simulink model "realtime_maglev_model"  (R2013a)
settings: Solver=ode45  StartTime=0.0  StopTime=10.0  RelTol=1e-3
undefined symbols (not defined in the file or in its folder): Advantech, PCI
libraries: rtwinlib x2, simulink x2
settings Model: Creator=Levitador  LastModifiedBy=Levitador

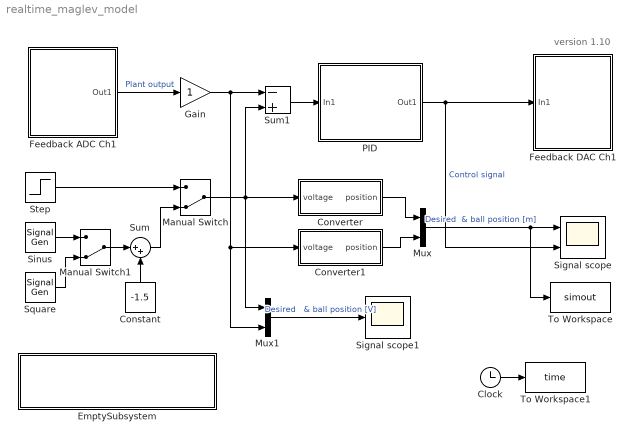
== system realtime_maglev_model ==
  note: version 1.10
  Clock : Clock
  Constant : Constant  Value=-1.5
  Converter : Subsystem
  Converter1 : Subsystem
  EmptySubsystem : Subsystem
      mask Display:
      | image(imread('FB-inst-blue2.jpg'))
      | disp('\n\nFeedback Instruments Limited')
  Feedback ADC Ch1 : Subsystem  mask{Tsamp=0.001}
      mask prompts: Tsamp "Sampling time"
      mask Display:
      | image(imread('bckg.bmp'))
      | disp('PCI1711 \n Lab I/O Board \n\n Feedback  ADC')
  Feedback DAC Ch1 : Subsystem  mask(DAC Unit for Feedback Experiments){st=0.001, ch=1}
      mask prompts: st "Sample Time"; ch "Output Channel"
      mask help:
      | Digital to Analog Output  for Feedback Experiments
      | using Advantech PCI1711  I/O board
      mask Display:
      | image(imread('bckg.bmp'))
      | disp('PCI1711 \n Lab I/O Board \n\n Feedback  DAC')
  Gain : Gain
  Manual Switch : ManualSwitch  CurrentSetting=0
  Manual Switch1 : ManualSwitch  CurrentSetting=0
  Mux : Mux  Inputs=2
  Mux1 : Mux  Inputs=2
  PID : Subsystem  mask{Kp=4, Ki=2.3, Kd=0.2}
      mask Display:
      | image(imread('bckg.bmp'))
      | disp('PID')
  Signal scope : Scope  NumInputPorts=2
      settings: TimeRange=100  YMin=0.0135~-175  YMax=0.0215~175  MaxDataPoints=500000
      mask Display: image(imread('scope.jpg'))
  Signal scope1 : Scope
      settings: TimeRange=100  YMin=-2.4  YMax=-0.7  MaxDataPoints=500000
      mask Display: image(imread('scope.jpg'))
  Sinus : SignalGenerator  Amplitude=0.5  Frequency=0.5
  Square : SignalGenerator  WaveForm=square  Amplitude=0.4  Frequency=0.1
  Step : Step  Time=10  Before=-1  After=-2  SampleTime=0
  Sum : Sum  Inputs=|++
  Sum1 : Sum  Inputs=-+  SaturateOnIntegerOverflow=on  InputSameDT=on  OutDataTypeStr=Inherit: Same as first input
  To Workspace : ToWorkspace  VariableName=simout  SampleTime=0.01
  To Workspace1 : ToWorkspace  VariableName=time  SampleTime=0.01
  wires:
  Sum1/1 -> PID/1(In1)
  Feedback ADC Ch1/1(Out1) -> Gain/1  "Plant output"
  PID/1(Out1) -> Feedback DAC Ch1/1(In1), Signal scope/2  "Control signal"
  Step/1 -> Manual Switch/1
  Square/1 -> Manual Switch1/2
  Sinus/1 -> Manual Switch1/1
  Manual Switch/1 -> Sum1/2, Converter/1(voltage), Mux1/1
  Manual Switch1/1 -> Sum/1
  Constant/1 -> Sum/2
  Sum/1 -> Manual Switch/2
  Mux/1 -> Signal scope/1, To Workspace/1  "Desired  & ball position [m]"
  Converter/1(position) -> Mux/1
  Converter1/1(position) -> Mux/2
  Mux1/1 -> Signal scope1/1  "Desired   & ball position [V]"
  Clock/1 -> To Workspace1/1
  Gain/1 -> Sum1/1, Converter1/1(voltage), Mux1/2

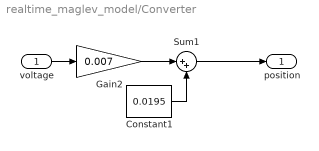
== system realtime_maglev_model/Converter ==
  voltage : Inport
  Constant1 : Constant  Value=0.0195
  Gain2 : Gain  Gain=0.007
  Sum1 : Sum  Inputs=|++
  position : Outport
  wires:
  Gain2/1 -> Sum1/1
  Constant1/1 -> Sum1/2
  voltage/1 -> Gain2/1
  Sum1/1 -> position/1

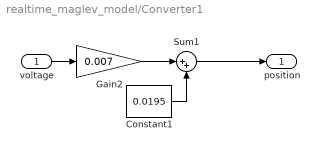
== system realtime_maglev_model/Converter1 ==
  voltage : Inport
  Constant1 : Constant  Value=0.0195
  Gain2 : Gain  Gain=0.007
  Sum1 : Sum  Inputs=|++
  position : Outport
  wires:
  Sum1/1 -> position/1
  voltage/1 -> Gain2/1
  Constant1/1 -> Sum1/2
  Gain2/1 -> Sum1/1

== system realtime_maglev_model/EmptySubsystem ==

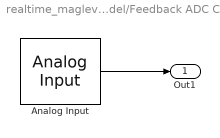
== system realtime_maglev_model/Feedback ADC Ch1 ==
  Analog Input : rtwinlib/Analog Input  SampleTime=Tsamp  MaxMissedTicks=10  ShowMissedTicks=off  YieldWhenWaiting=off  DrvName=Advantech/PCI-1711  DrvAddress=4294967295  DrvOptions=zeros(1,0)  Channels=11  RangeMode=1  VoltRange=1  DataType=1
      settings: AttributesFormatString=Advantech\nPCI-1711 [auto]
  Out1 : Outport
  wires:
  Analog Input/1 -> Out1/1

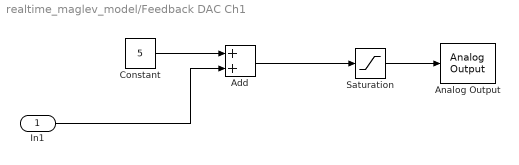
== system realtime_maglev_model/Feedback DAC Ch1 ==
  In1 : Inport
  Add : Sum  OutDataTypeStr=Inherit: Same as first input
  Analog Output : rtwinlib/Analog Output  SampleTime=st  MaxMissedTicks=10  ShowMissedTicks=off  YieldWhenWaiting=off  DrvName=Advantech/PCI-1711  DrvAddress=4294967295  DrvOptions=zeros(1,0)  Channels=ch  RangeMode=1  VoltRange=2  InitialValue=5  FinalValue=5
      settings: AttributesFormatString=Advantech\nPCI-1711 [auto]
  Constant : Constant  Value=5
  Saturation : Saturate  UpperLimit=10  LowerLimit=0
  wires:
  In1/1 -> Add/2
  Constant/1 -> Add/1
  Saturation/1 -> Analog Output/1
  Add/1 -> Saturation/1

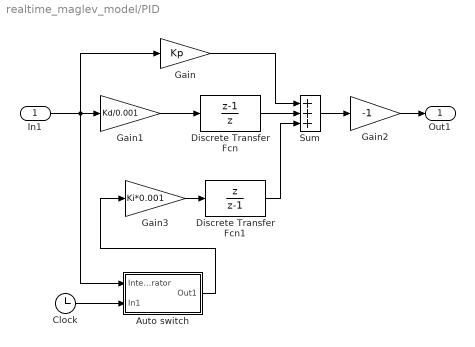
== system realtime_maglev_model/PID ==
  In1 : Inport
  Auto switch : Subsystem
  Clock : Clock
  Discrete Transfer Fcn : DiscreteTransferFcn  Numerator=[1 -1]  Denominator=[1 0]  SampleTime=0.001
  Discrete Transfer Fcn1 : DiscreteTransferFcn  Numerator=[1 0]  Denominator=[1 -1]  SampleTime=0.001
  Gain : Gain  Gain=Kp  SampleTime=0.001
  Gain1 : Gain  Gain=Kd/0.001  SampleTime=0.001
  Gain2 : Gain  Gain=-1
  Gain3 : Gain  Gain=Ki*0.001  SampleTime=0.001
  Sum : Sum  Inputs=+++
  Out1 : Outport
  wires:
  In1/1 -> Gain/1, Gain1/1, Auto switch/1(Integrator)
  Gain/1 -> Sum/1
  Sum/1 -> Gain2/1
  Gain2/1 -> Out1/1
  Discrete Transfer Fcn/1 -> Sum/2
  Gain1/1 -> Discrete Transfer Fcn/1
  Discrete Transfer Fcn1/1 -> Sum/3
  Clock/1 -> Auto switch/2(In1)
  Auto switch/1(Out1) -> Gain3/1
  Gain3/1 -> Discrete Transfer Fcn1/1

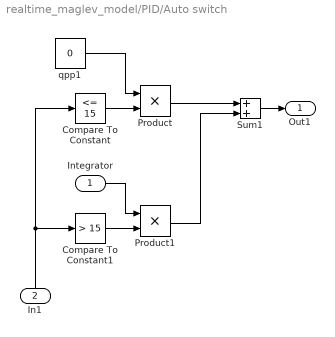
== system realtime_maglev_model/PID/Auto switch ==
  Integrator : Inport
  In1 : Inport  Port=2
  Compare To Constant : simulink/Logic and Bit Operations/Compare To Constant  relop=<=  const=15  OutDataTypeStr=boolean  ZeroCross=off
  Compare To Constant1 : simulink/Logic and Bit Operations/Compare To Constant  relop=>  const=15  OutDataTypeStr=boolean  ZeroCross=off
  Product : Product  RndMeth=Zero
  Product1 : Product  RndMeth=Zero
  Sum1 : Sum
  qpp1 : Constant  Value=0
  Out1 : Outport
  wires:
  Integrator/1 -> Product1/1
  Sum1/1 -> Out1/1
  In1/1 -> Compare To Constant1/1, Compare To Constant/1
  Product1/1 -> Sum1/2
  Compare To Constant1/1 -> Product1/2
  Product/1 -> Sum1/1
  qpp1/1 -> Product/1
  Compare To Constant/1 -> Product/2
